simulink model "Spindel_P_Var"  (Simulink 7.6)
settings: Solver=ode45  StartTime=0.0  StopTime=SimulTime  RelTol=1e-3
values from neighbouring files (symbols this model uses):
  Ein = 1    [ParamtersSpindel_P_Var.m]
  MaxDrehmoment = 265    [ParamtersSpindel_P_Var.m]
  MaxDrehzahl = 6500    [ParamtersSpindel_P_Var.m]
  PR = 5    [ParamtersSpindel_P_Var.m]
  radius = 0.15    [ParamtersSpindel_P_Var.m]
undefined symbols (not defined in the file or in its folder): Job, m, Spindel
settings Model: Creator=Coni  LastModifiedBy=conid

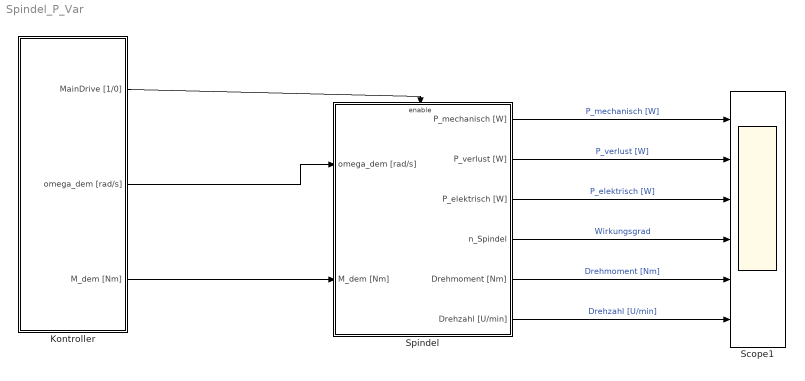
== system Spindel_P_Var ==
  Kontroller : Subsystem
  Scope1 : Scope  NumInputPorts=6
      settings: TimeRange=100  YMin=0~-5000~-2000~-0.1~-5~-5  YMax=16000~30000~14000~0.9~5~5  SaveName=Scp_MainDrive
  Spindel : Subsystem  TreatAsAtomicUnit=on
  wires:
  Kontroller/2(omega_dem [rad/s]) -> Spindel/1(omega_dem [rad/s])
  Kontroller/3(M_dem [Nm]) -> Spindel/2(M_dem [Nm])
  Kontroller/1(MainDrive [1/0]) -> Spindel/Enable
  Spindel/4(n_Spindel) -> Scope1/4  "Wirkungsgrad"
  Spindel/2(P_verlust [W]) -> Scope1/2  "P_verlust [W]"
  Spindel/3(P_elektrisch [W]) -> Scope1/3  "P_elektrisch [W]"
  Spindel/5(Drehmoment [Nm]) -> Scope1/5  "Drehmoment [Nm]"
  Spindel/6(Drehzahl [U/min]) -> Scope1/6  "Drehzahl [U/min]"
  Spindel/1(P_mechanisch [W]) -> Scope1/1  "P_mechanisch [W]"

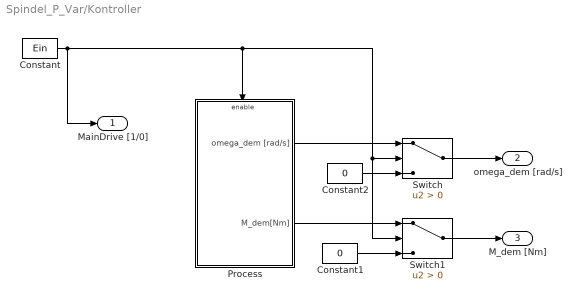
== system Spindel_P_Var/Kontroller ==
  Constant : Constant  Value=Ein
  Constant1 : Constant  Value=0
  Constant2 : Constant  Value=0
  Process : Subsystem  TreatAsAtomicUnit=on
  Switch : Switch  Criteria=u2 > Threshold
  Switch1 : Switch  Criteria=u2 > Threshold
  MainDrive [1/0] : Outport
  omega_dem [rad/s] : Outport  Port=2
  M_dem [Nm] : Outport  Port=3
  wires:
  Constant/1 -> Process/Enable, Switch1/2, Switch/2, MainDrive [1/0]/1
  Process/1(omega_dem [rad/s]) -> Switch/1
  Process/2(M_dem[Nm]) -> Switch1/1
  Constant1/1 -> Switch1/3
  Switch/1 -> omega_dem [rad/s]/1
  Switch1/1 -> M_dem [Nm]/1
  Constant2/1 -> Switch/3

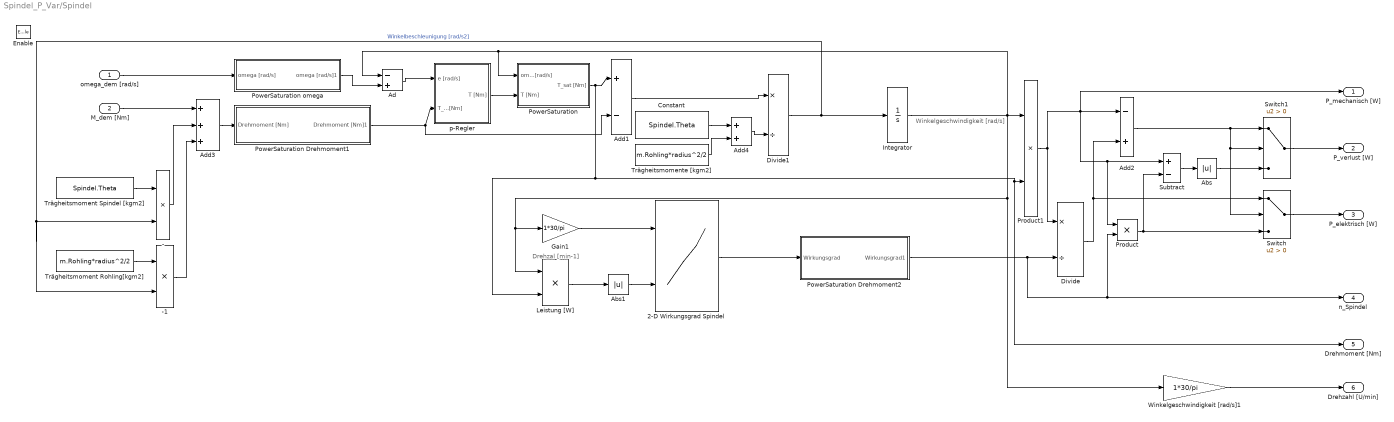
== system Spindel_P_Var/Spindel ==
  note: Winkelgeschwindigkeit [rad/s]
  note: Drehzal [min-1]
  omega_dem [rad/s] : Inport
  M_dem [Nm] : Inport  Port=2
  Enable : EnablePort
  - : Product  RndMeth=Zero
  -1 : Product  RndMeth=Zero
  2-D Wirkungsgrad Spindel : Lookup_n-D  BreakpointsForDimension1=Spindel.Tabelleomega  BreakpointsForDimension2=Spindel.TabelleM  Table=Spindel.Tabelleeta  InterpMethod=Cubic spline  RndMeth=Simplest  InputSameDT=on
  Abs : Abs
  Abs1 : Abs
  Ad : Sum  Inputs=-+
  Add1 : Sum  Inputs=+-
  Add2 : Sum  Inputs=-+
  Add3 : Sum  Inputs=+++
  Add4 : Sum
  Constant : Constant  Value=Spindel.Theta
  Divide : Product  Inputs=*/
  Divide1 : Product  Inputs=*/
  Gain1 : Gain  Gain=1*30/pi
  Integrator : Integrator
  Leistung [W] : Product  RndMeth=Zero
  PowerSaturation : Subsystem  TreatAsAtomicUnit=on
  PowerSaturation Drehmoment1 : Subsystem  TreatAsAtomicUnit=on
  PowerSaturation Drehmoment2 : Subsystem  TreatAsAtomicUnit=on
  PowerSaturation omega : Subsystem  TreatAsAtomicUnit=on
  Product : Product  RndMeth=Zero
  Product1 : Product  RndMeth=Zero
  Subtract : Sum  Inputs=+-
  Switch : Switch  Criteria=u2 > Threshold
  Switch1 : Switch  Criteria=u2 > Threshold
  Trägheitsmoment Rohling[kgm2] : Constant  Value=m.Rohling*radius^2/2
  Trägheitsmoment Spindel [kgm2] : Constant  Value=Spindel.Theta
  Trägheitsmomente [kgm2] : Constant  Value=m.Rohling*radius^2/2
  Winkelgeschwindigkeit [rad/s]1 : Gain  Gain=1*30/pi
  p-Regler : Subsystem  TreatAsAtomicUnit=on
  P_mechanisch [W] : Outport
  P_verlust [W] : Outport  Port=2
  P_elektrisch [W] : Outport  Port=3
  n_Spindel : Outport  Port=4
  Drehmoment [Nm] : Outport  Port=5
  Drehzahl [U/min] : Outport  Port=6
  wires:
  Ad/1 -> p-Regler/1(e [rad/s])
  p-Regler/1(T [Nm]) -> PowerSaturation/2(T [Nm])
  PowerSaturation/1(T_sat [Nm]) -> Leistung [W]/2, Product1/2, Drehmoment [Nm]/1, Add1/1
  Integrator/1 -> Product1/1, Ad/1, PowerSaturation/1(omega [rad/s]), Leistung [W]/1, Gain1/1, Winkelgeschwindigkeit [rad/s]1/1
  Product1/1 -> Divide/1, Add2/1, P_mechanisch [W]/1, Subtract/1, Product/1
  Divide/1 -> Add2/2, Switch/1
  Gain1/1 -> 2-D Wirkungsgrad Spindel/1
  Trägheitsmoment Spindel [kgm2]/1 -> -/1
  M_dem [Nm]/1 -> Add3/1
  -/1 -> Add3/2
  -1/1 -> Add3/3
  Trägheitsmoment Rohling[kgm2]/1 -> -1/1
  Add1/1 -> Divide1/1
  Divide1/1 -> Integrator/1, -1/2, -/2  "Winkelbeschleunigung [rad/s2]"
  Add4/1 -> Divide1/2
  Constant/1 -> Add4/1
  Trägheitsmomente [kgm2]/1 -> Add4/2
  Switch1/1 -> P_verlust [W]/1
  Switch/1 -> P_elektrisch [W]/1
  Add2/1 -> Switch1/1, Switch1/2, Switch/2
  Product/1 -> Subtract/2, Switch/3
  Subtract/1 -> Abs/1
  Abs/1 -> Switch1/3
  Abs1/1 -> 2-D Wirkungsgrad Spindel/2
  Leistung [W]/1 -> Abs1/1
  Winkelgeschwindigkeit [rad/s]1/1 -> Drehzahl [U/min]/1
  Add3/1 -> PowerSaturation Drehmoment1/1(Drehmoment [Nm])
  PowerSaturation Drehmoment1/1(Drehmoment [Nm]1) -> Add1/2, p-Regler/2(T_dem [Nm])
  omega_dem [rad/s]/1 -> PowerSaturation omega/1(omega [rad/s])
  PowerSaturation omega/1(omega [rad/s]1) -> Ad/2
  2-D Wirkungsgrad Spindel/1 -> PowerSaturation Drehmoment2/1(Wirkungsgrad)
  PowerSaturation Drehmoment2/1(Wirkungsgrad1) -> Divide/2, n_Spindel/1, Product/2

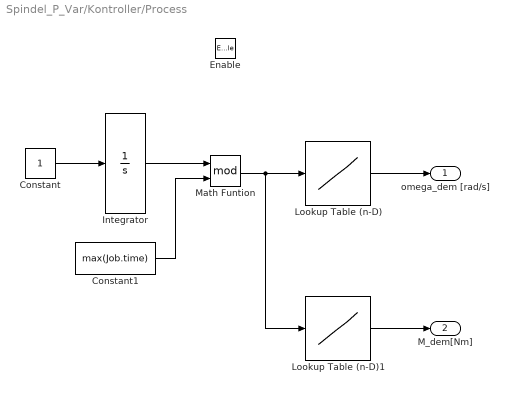
== system Spindel_P_Var/Kontroller/Process ==
  Enable : EnablePort
  Constant : Constant
  Constant1 : Constant  Value=max(Job.time)
  Integrator : Integrator
  Lookup Table (n-D) : Lookup_n-D  NumberOfTableDimensions=1  BreakpointsForDimension1=Job.time  Table=Job.omega_dem  InterpMethod=None - Flat  ExtrapMethod=Cubic spline  InputSameDT=on
  Lookup Table (n-D)1 : Lookup_n-D  NumberOfTableDimensions=1  BreakpointsForDimension1=Job.time  Table=Job.M_dem  InterpMethod=None - Flat  InputSameDT=on
  Math Funtion : Math  Operator=mod  SaturateOnIntegerOverflow=on
  omega_dem [rad/s] : Outport
  M_dem[Nm] : Outport  Port=2
  wires:
  Constant/1 -> Integrator/1
  Integrator/1 -> Math Funtion/1
  Math Funtion/1 -> Lookup Table (n-D)/1, Lookup Table (n-D)1/1
  Lookup Table (n-D)/1 -> omega_dem [rad/s]/1
  Lookup Table (n-D)1/1 -> M_dem[Nm]/1
  Constant1/1 -> Math Funtion/2

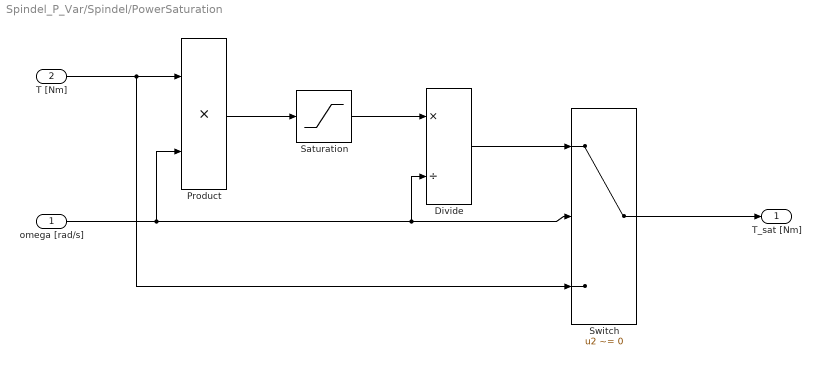
== system Spindel_P_Var/Spindel/PowerSaturation ==
  omega [rad/s] : Inport
  T [Nm] : Inport  Port=2
  Divide : Product  Inputs=*/
  Product : Product  RndMeth=Zero
  Saturation : Saturate  UpperLimit=Spindel.Pmax  LowerLimit=-Spindel.Pmax
  Switch : Switch  Criteria=u2 ~= 0
  T_sat [Nm] : Outport
  wires:
  Product/1 -> Saturation/1
  Saturation/1 -> Divide/1
  Divide/1 -> Switch/1
  Switch/1 -> T_sat [Nm]/1
  T [Nm]/1 -> Product/1, Switch/3
  omega [rad/s]/1 -> Switch/2, Divide/2, Product/2

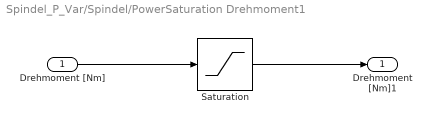
== system Spindel_P_Var/Spindel/PowerSaturation Drehmoment1 ==
  Drehmoment [Nm] : Inport
  Saturation : Saturate  UpperLimit=MaxDrehmoment  LowerLimit=-MaxDrehmoment  ZeroCross=off
  Drehmoment [Nm]1 : Outport
  wires:
  Drehmoment [Nm]/1 -> Saturation/1
  Saturation/1 -> Drehmoment [Nm]1/1

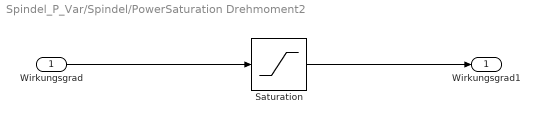
== system Spindel_P_Var/Spindel/PowerSaturation Drehmoment2 ==
  Wirkungsgrad : Inport
  Saturation : Saturate  UpperLimit=0.95  LowerLimit=0.1  ZeroCross=off
  Wirkungsgrad1 : Outport
  wires:
  Wirkungsgrad/1 -> Saturation/1
  Saturation/1 -> Wirkungsgrad1/1

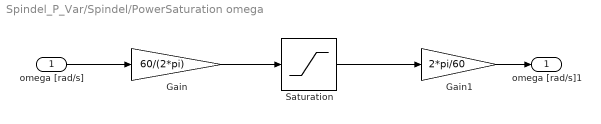
== system Spindel_P_Var/Spindel/PowerSaturation omega ==
  omega [rad/s] : Inport
  Gain : Gain  Gain=60/(2*pi)
  Gain1 : Gain  Gain=2*pi/60
  Saturation : Saturate  UpperLimit=MaxDrehzahl  LowerLimit=0  ZeroCross=off
  omega [rad/s]1 : Outport
  wires:
  Saturation/1 -> Gain1/1
  omega [rad/s]/1 -> Gain/1
  Gain1/1 -> omega [rad/s]1/1
  Gain/1 -> Saturation/1

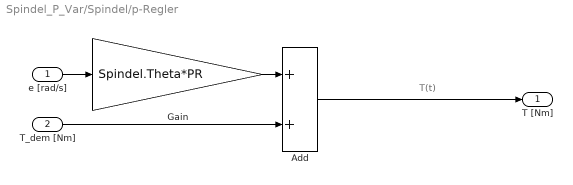
== system Spindel_P_Var/Spindel/p-Regler ==
  note: T(t)
  e [rad/s] : Inport
  T_dem [Nm] : Inport  Port=2
  Add : Sum
  Gain : Gain  Gain=Spindel.Theta*PR
  T [Nm] : Outport
  wires:
  Add/1 -> T [Nm]/1
  T_dem [Nm]/1 -> Add/2
  Gain/1 -> Add/1
  e [rad/s]/1 -> Gain/1
